simulink model "cross_track_error"  (Simulink 7.9)
settings: Solver=ode45  StartTime=0.0  StopTime=10  RelTol=1e-3
values from neighbouring files (symbols this model uses):
  A = 0.002    [params.m]
  D = 5    [params.m]
  v = 100    [params.m]
libraries: simulink x3
settings Model: Creator=dave  LastModifiedBy=dave

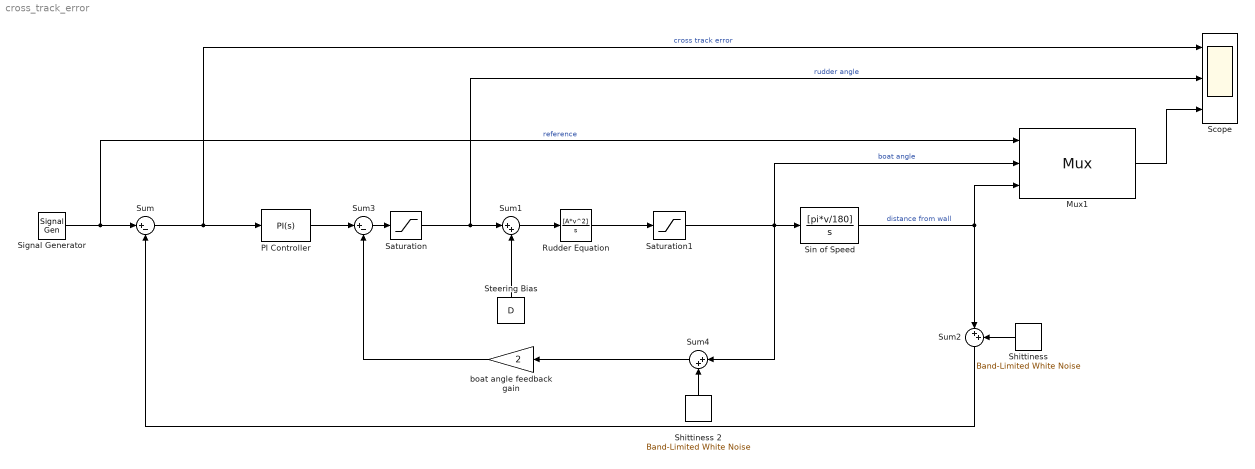
== system cross_track_error ==
  Mux1 : Mux  Inputs=3
      settings: DisplayOption=signals
  PI Controller : simulink/Continuous/PID Controller  Controller=PI  TimeDomain=Continuous-time  SampleTime=1  IntegratorMethod=Forward Euler  FilterMethod=Forward Euler  Form=Parallel  P=2.6  I=0.3  D=0  N=7.02962681019428  InitialConditionSource=internal  InitialConditionForIntegrator=0  InitialConditionForFilter=0  ExternalReset=none  LimitOutput=off  UpperSaturationLimit=inf  LowerSaturationLimit=-inf  LinearizeAsGain=off  AntiWindupMode=none  Kb=1  TrackingMode=off  Kt=1  PParamMin=[]  PParamMax=[]  IParamMin=[]  IParamMax=[]  DParamMin=[]  DParamMax=[]  NParamMin=[]  NParamMax=[]  KbParamMin=[]  KbParamMax=[]  KtParamMin=[]  KtParamMax=[]  POutMin=[]  POutMax=[]  IOutMin=[]  IOutMax=[]  DOutMin=[]  DOutMax=[]  NOutMin=[]  NOutMax=[]  KbOutMin=[]  KbOutMax=[]  KtOutMin=[]  KtOutMax=[]  IntegratorOutMin=[]  IntegratorOutMax=[]  FilterOutMin=[]  FilterOutMax=[]  SumOutMin=[]  SumOutMax=[]  SumI1OutMin=[]  SumI1OutMax=[]  SumI2OutMin=[]  SumI2OutMax=[]  SumI3OutMin=[]  SumI3OutMax=[]  SumDOutMin=[]  SumDOutMax=[]  SaturationOutMin=[]  SaturationOutMax=[]  IntegratorContinuousStateAttributes=''  IntegratorStateMustResolveToSignalObject=off  IntegratorRTWStateStorageClass=Auto  FilterContinuousStateAttributes=''  FilterStateMustResolveToSignalObject=off  FilterRTWStateStorageClass=Auto
  Rudder Equation : TransferFcn  Numerator=[A*v^2]  Denominator=[1 0]
  Saturation : Saturate  UpperLimit=25  LowerLimit=-25
  Saturation1 : Saturate  UpperLimit=35  LowerLimit=-35
  Scope : Scope  NumInputPorts=3
      settings: ShowLegends=on  TimeRange=10  YMin=-60~-30~-30  YMax=40~20~30
  Shittiness : simulink/Sources/Band-Limited White Noise  Cov=[0.05]  Ts=0.05  seed=[23341]
  Shittiness 2 : simulink/Sources/Band-Limited White Noise  Cov=[0.05]  Ts=0.05  seed=[2352351]
  Signal Generator : SignalGenerator  WaveForm=square  Amplitude=20  Frequency=0.25
  Sin of Speed : TransferFcn  Numerator=[pi*v/180]  Denominator=[1 0]
  Steering Bias : Constant  Value=D
  Sum : Sum  Inputs=|+-
  Sum1 : Sum  Inputs=|++
  Sum2 : Sum  Inputs=|++
  Sum3 : Sum  Inputs=|+-
  Sum4 : Sum  Inputs=|++
  boat angle feedback gain : Gain  Gain=2
  wires:
  Sum/1 -> PI Controller/1, Scope/1  "cross track error"
  Signal Generator/1 -> Sum/1, Mux1/1  "reference"
  Mux1/1 -> Scope/3
  Sin of Speed/1 -> Mux1/3, Sum2/1  "distance from wall"
  Saturation/1 -> Scope/2, Sum1/1  "rudder angle"
  PI Controller/1 -> Sum3/1
  Sum3/1 -> Saturation/1
  boat angle feedback gain/1 -> Sum3/2
  Steering Bias/1 -> Sum1/2
  Sum1/1 -> Rudder Equation/1
  Saturation1/1 -> Sin of Speed/1, Mux1/2, Sum4/1  "boat angle"
  Rudder Equation/1 -> Saturation1/1
  Sum4/1 -> boat angle feedback gain/1
  Shittiness 2/1 -> Sum4/2
  Sum2/1 -> Sum/2
  Shittiness/1 -> Sum2/2
